simulink model "Copy_of_lab_model"  (Simulink 9.2)
settings: Solver=ode45  StartTime=0.0  StopTime=1  RelTol=1e-3  EnableMultiTasking=on
values from neighbouring files (symbols this model uses):
  A0 = 2.5    [lab_vars.m]
  J = Jco+Jm    (= 10.2)    [lab_vars.m]
  Kcur_fdb = round(kcs*kadc)    [lab_vars.m]
  kcur_i = 5    [lab_vars.m]
  kcur_p = 10    [lab_vars.m]
  Ke = Km    (= 5)    [lab_vars.m]
  Kf = 0.01    [lab_vars.m]
  Km = 5    [lab_vars.m]
  Kpwc = Un/Uc    (= 2.5)    [lab_vars.m]
  Ksi = 0.5    [lab_vars.m]
  Kspd_fdb = round(kps_int*Ts,1)    [lab_vars.m]
  kspd_p = 10    [lab_vars.m]
  R = 5    [lab_vars.m]
  tau_filt = 1/W0    (= 0.01)    [lab_vars.m]
  Te = 0.0005    [lab_vars.m]
  Tf = 0.10    (= 0.1)    [lab_vars.m]
  Tpwc = 0.002    [lab_vars.m]
  W0 = 100    [lab_vars.m]
settings Model: Creator=Student  LastModifiedBy=murad
settings DataIOCC: LimitDataPoints=off  SaveFormat=StructureWithTime
settings DebuggingCC: UnderspecifiedInitializationDetection=Simplified  MergeDetectMultiDrivingBlocksExec=error  StateNameClashWarn=none
settings HardwareCC: ProdIntDivRoundTo=Zero  ProdEndianess=LittleEndian  ProdHWDeviceType=Specified

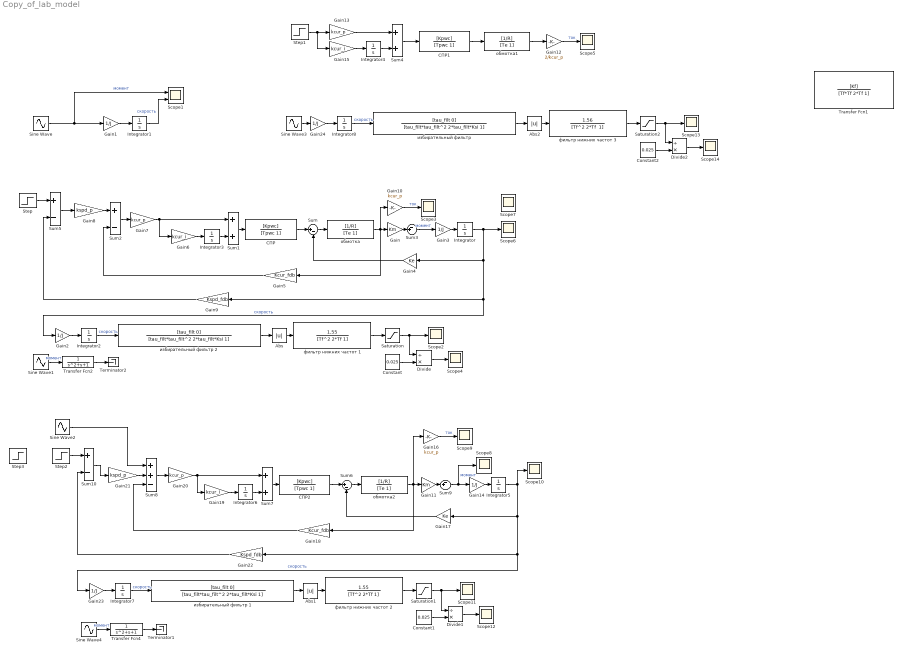
== system Copy_of_lab_model ==
  Abs : Abs
  Abs1 : Abs
  Abs2 : Abs
  Constant : Constant  Value=0.025
  Constant1 : Constant  Value=0.025
  Constant2 : Constant  Value=0.025
  Divide : Product  Inputs=/*
  Divide1 : Product  Inputs=/*
  Divide2 : Product  Inputs=/*
  Gain : Gain  Gain=Km
  Gain{1..3,14,23..24} (6 alike) : Gain  Gain=1/J
  Gain{7,10,13,16,20} (5 alike) : Gain  Gain=kcur_p
  Gain11 : Gain  Gain=Km
  Gain12 : Gain  Gain=2/kcur_p
  Gain15 : Gain  Gain=kcur_i
  Gain17 : Gain  Gain=Ke
  Gain18 : Gain  Gain=Kcur_fdb
  Gain19 : Gain  Gain=kcur_i
  Gain21 : Gain  Gain=kspd_p
  Gain22 : Gain  Gain=Kspd_fdb
  Gain4 : Gain  Gain=Ke
  Gain5 : Gain  Gain=Kcur_fdb
  Gain6 : Gain  Gain=kcur_i
  Gain8 : Gain  Gain=kspd_p
  Gain9 : Gain  Gain=Kspd_fdb
  Integrator{,1..8} (9 alike) : Integrator
  Saturation : Saturate  UpperLimit=0.025  LowerLimit=0.00025
  Saturation1 : Saturate  UpperLimit=0.025  LowerLimit=0.00025
  Saturation2 : Saturate  UpperLimit=0.025  LowerLimit=0.00025
  Scope1 : Scope  NumInputPorts=2
  Scope{2..14} (13 alike) : Scope
  Sine Wave : Sin  Amplitude=A0  Frequency=W0  SampleTime=0
  Sine Wave1 : Sin  Frequency=200000  SampleTime=0
  Sine Wave2 : Sin  Amplitude=A0*50  Frequency=W0  SampleTime=0
  Sine Wave3 : Sin  Amplitude=A0  Frequency=W0  SampleTime=0
  Sine Wave4 : Sin  Frequency=200000  SampleTime=0
  Step{,1..3} (4 alike) : Step  Time=0  After=A0  SampleTime=0
  Sum : Sum  Inputs=|+-
  Sum1 : Sum
  Sum10 : Sum  Inputs=+-
  Sum2 : Sum  Inputs=+-
  Sum3 : Sum  Inputs=-+|
  Sum4 : Sum
  Sum5 : Sum  Inputs=+-
  Sum6 : Sum  Inputs=|+-
  Sum7 : Sum
  Sum8 : Sum  Inputs=++-
  Sum9 : Sum  Inputs=-+|
  Terminator1 : Terminator
  Terminator2 : Terminator
  Transfer Fcn1 : TransferFcn  Numerator=[Kf]  Denominator=[Tf*Tf 2*Tf 1]
  Transfer Fcn2 : TransferFcn  Numerator=[ 1]  Denominator=[1 1 1]
  Transfer Fcn4 : TransferFcn  Numerator=[ 1]  Denominator=[1 1 1]
  СПР : TransferFcn  Numerator=[Kpwc]  Denominator=[Tpwc 1]
  СПР1 : TransferFcn  Numerator=[Kpwc]  Denominator=[Tpwc 1]
  СПР2 : TransferFcn  Numerator=[Kpwc]  Denominator=[Tpwc 1]
  "избирательный фильтр " : TransferFcn  Numerator=[tau_filt 0]  Denominator=[tau_filt*tau_filt^2 2*tau_filt*Ksi 1]
  избирательный фильтр 1 : TransferFcn  Numerator=[tau_filt 0]  Denominator=[tau_filt*tau_filt^2 2*tau_filt*Ksi 1]
  избирательный фильтр 2 : TransferFcn  Numerator=[tau_filt 0]  Denominator=[tau_filt*tau_filt^2 2*tau_filt*Ksi 1]
  обмотка : TransferFcn  Numerator=[1/R]  Denominator=[Te 1]
  обмотка1 : TransferFcn  Numerator=[1/R]  Denominator=[Te 1]
  обмотка2 : TransferFcn  Numerator=[1/R]  Denominator=[Te 1]
  фильтр нижних частот 1 : TransferFcn  Numerator=[1.55]  Denominator=[Tf^2 2*Tf 1]
  фильтр нижних частот 2 : TransferFcn  Numerator=[1.55]  Denominator=[Tf^2 2*Tf 1]
  фильтр нижних частот 3 : TransferFcn  Numerator=[1.56]  Denominator="[Tf^2 2*Tf  1]"
  wires:
  Sine Wave/1 -> Gain1/1, Scope1/1  "момент"
  Gain1/1 -> Integrator1/1
  Integrator1/1 -> Scope1/2  "скорость"
  Abs/1 -> фильтр нижних частот 1/1
  Integrator2/1 -> избирательный фильтр 2/1  "скорость"
  Gain2/1 -> Integrator2/1
  Integrator/1 -> Scope6/1, Gain2/1, Gain9/1, Gain4/1  "скорость"
  фильтр нижних частот 1/1 -> Saturation/1
  Divide/1 -> Scope4/1
  Constant/1 -> Divide/2
  избирательный фильтр 2/1 -> Abs/1
  Saturation/1 -> Divide/1, Scope2/1
  Gain4/1 -> Sum/2
  Sum/1 -> обмотка/1
  Step/1 -> Sum5/1
  Gain9/1 -> Sum5/2
  Sum3/1 -> Gain3/1  "момент"
  Gain3/1 -> Integrator/1
  Sum1/1 -> СПР/1
  Gain7/1 -> Gain6/1, Sum1/1
  Gain/1 -> Sum3/2
  СПР/1 -> Sum/1
  Integrator3/1 -> Sum1/2
  Gain5/1 -> Sum2/2
  Sum5/1 -> Gain8/1
  Gain6/1 -> Integrator3/1
  Sum2/1 -> Gain7/1
  обмотка/1 -> Gain10/1, Gain5/1, Gain/1
  Gain8/1 -> Sum2/1
  Gain10/1 -> Scope3/1  "ток"
  Gain12/1 -> Scope5/1  "ток"
  Gain13/1 -> Sum4/1
  Step1/1 -> Gain15/1, Gain13/1
  Gain15/1 -> Integrator4/1
  Sum4/1 -> СПР1/1
  СПР1/1 -> обмотка1/1
  Integrator4/1 -> Sum4/2
  обмотка1/1 -> Gain12/1
  Sine Wave2/1 -> Sum8/1
  Sum9/1 -> Scope8/1, Gain14/1  "момент"
  СПР2/1 -> Sum6/1
  Sum6/1 -> обмотка2/1
  Gain22/1 -> Sum10/2
  обмотка2/1 -> Gain16/1, Gain18/1, Gain11/1
  Gain21/1 -> Sum8/2
  Sum7/1 -> СПР2/1
  Sum8/1 -> Gain20/1
  Gain11/1 -> Sum9/2
  Step2/1 -> Sum10/1
  Gain18/1 -> Sum8/3
  Integrator6/1 -> Sum7/2
  Gain20/1 -> Gain19/1, Sum7/1
  Gain17/1 -> Sum6/2
  Sum10/1 -> Gain21/1
  Gain16/1 -> Scope9/1  "ток"
  Gain14/1 -> Integrator5/1
  Gain19/1 -> Integrator6/1
  фильтр нижних частот 2/1 -> Saturation1/1
  Saturation1/1 -> Divide1/1, Scope11/1
  Integrator7/1 -> избирательный фильтр 1/1  "скорость"
  Constant1/1 -> Divide1/2
  Sine Wave4/1 -> Transfer Fcn4/1  "момент"
  Transfer Fcn4/1 -> Terminator1/1
  Gain23/1 -> Integrator7/1
  Integrator5/1 -> Scope10/1, Gain23/1, Gain22/1, Gain17/1  "скорость"
  Abs1/1 -> фильтр нижних частот 2/1
  Divide1/1 -> Scope12/1
  избирательный фильтр 1/1 -> Abs1/1
  фильтр нижних частот 3/1 -> Saturation2/1
  Saturation2/1 -> Divide2/1, Scope13/1
  Constant2/1 -> Divide2/2
  Gain24/1 -> Integrator8/1
  Abs2/1 -> фильтр нижних частот 3/1
  Divide2/1 -> Scope14/1
  Integrator8/1 -> "избирательный фильтр "/1  "скорость"
  "избирательный фильтр "/1 -> Abs2/1
  Sine Wave3/1 -> Gain24/1
  Transfer Fcn2/1 -> Terminator2/1
  Sine Wave1/1 -> Transfer Fcn2/1  "момент"
